simulink model "FiltroCuartoOrdenRealimentado"  (R2017a)
settings: Solver=ode23tb  StartTime=0.0  StopTime=25e-3  RelTol=0.1e-3
settings Model: Creator=Nicolas Zamora  LastModifiedBy=Nicolas Zamora

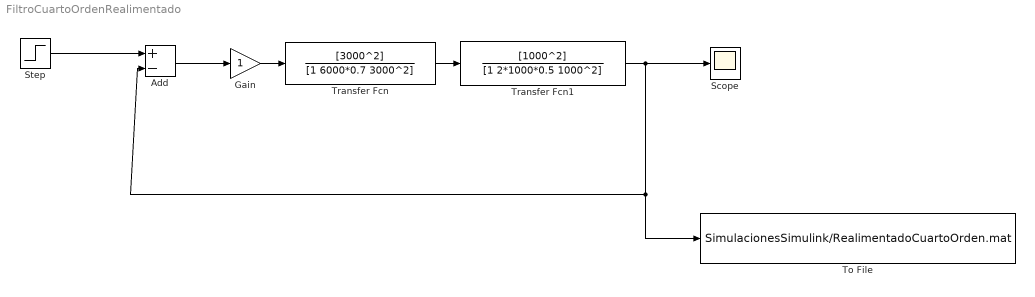
== system FiltroCuartoOrdenRealimentado ==
  Add : Sum  Inputs=+-
  Gain : Gain
  Scope : Scope
  Step : Step  Time=0  After=2  SampleTime=0
  To File : ToFile  Filename=SimulacionesSimulink/RealimentadoCuartoOrden.mat  MatrixName=datosmatlab
  Transfer Fcn : TransferFcn  Numerator=[3000^2]  Denominator=[1 6000*0.7 3000^2]
  Transfer Fcn1 : TransferFcn  Numerator=[1000^2]  Denominator=[1 2*1000*0.5 1000^2]
  wires:
  Step/1 -> Add/1
  Add/1 -> Gain/1
  Gain/1 -> Transfer Fcn/1
  Transfer Fcn/1 -> Transfer Fcn1/1
  Transfer Fcn1/1 -> To File/1, Add/2, Scope/1
